simulink model "VTOLAutopilotController (minhyun-purdue's conflicted copy 2025-07-07)"  (R2024b)
settings: configuration reference "VTOLConfiguration" (kept outside this file)
undefined symbols (not defined in the file): control, controlParams, ControlSampleTime, CriticalTiltAngle, DiscIntNeverNeededParam, dspblkCoreblockFVToolHelper, flightState, FSState, FWControlParams, FWTrimSpeed, gcbh, HoverMission, R_LOOKAHEAD, ReferenceFilterDen, ReferenceFilterNum, tilt_max, tiltIni, uavParam, VTOLcontrolGains, w_trim, WindDownRate
libraries: slpidlib x32, simulink x11, uavalgslib x7, simulink_extras x1
(part 1 of 6)
settings Model: DataDictionary=VTOLDynamicsData.sldd  Creator=The MathWorks, Inc.  LastModifiedBy=mhcho
settings ConfigSetRef: SourceName=VTOLConfiguration

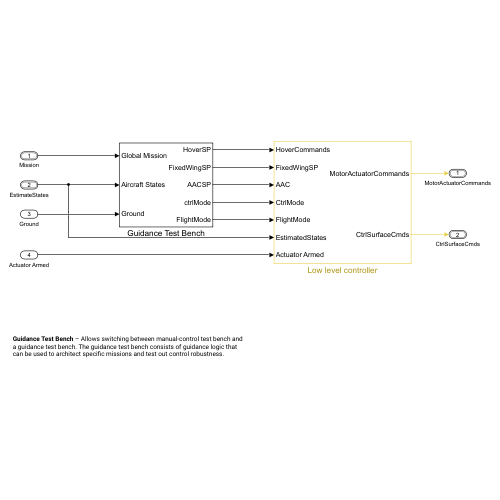
[thumbnail: Simulink's stored preview of the top-level diagram]
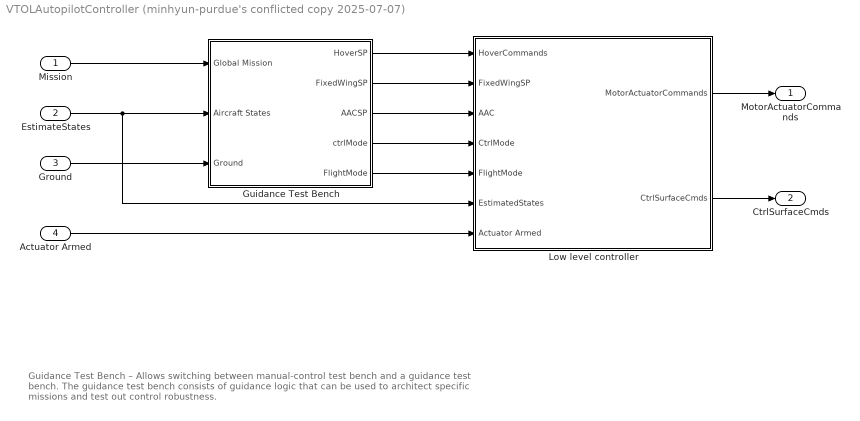
== system VTOLAutopilotController (minhyun-purdue's conflicted copy 2025-07-07) ==
  note: Guidance Test Bench – Allows switching between manual-control test bench and a guidance test bench. The guidance test bench consists of guidance logic that can be used to architect specific missions and test out control robustness.
  Mission : Inport  OutDataTypeStr=Bus: doubleUavPathManager  PortDimensions=length(HoverMission)  SampleTime=0.005  BusOutputAsStruct=on
  EstimateStates : Inport  Port=2  OutDataTypeStr=Bus: stateBus  BusOutputAsStruct=on
  Ground : Inport  Port=3  SampleTime=0.005
  Actuator Armed : Inport  Port=4
  Guidance Test Bench : Subsystem
  Low level controller : Subsystem
  MotorActuatorCommands : Outport  OutDataTypeStr=Bus: RotorCtrlBus  BusOutputAsStruct=on
  CtrlSurfaceCmds : Outport  Port=2  OutDataTypeStr=Bus: FixedWingCtrlBus  BusOutputAsStruct=on
  wires:
  Guidance Test Bench/1(HoverSP) -> Low level controller/1(HoverCommands)
  Guidance Test Bench/3(AACSP) -> Low level controller/3(AAC)
  Guidance Test Bench/5(FlightMode) -> Low level controller/5(FlightMode)
  Guidance Test Bench/4(ctrlMode) -> Low level controller/4(CtrlMode)
  EstimateStates/1 -> Guidance Test Bench/2(Aircraft States), Low level controller/6(EstimatedStates)
  Low level controller/1(MotorActuatorCommands) -> MotorActuatorCommands/1
  Mission/1 -> Guidance Test Bench/1(Global Mission)
  Guidance Test Bench/2(FixedWingSP) -> Low level controller/2(FixedWingSP)
  Low level controller/2(CtrlSurfaceCmds) -> CtrlSurfaceCmds/1
  Ground/1 -> Guidance Test Bench/3(Ground)
  Actuator Armed/1 -> Low level controller/7(Actuator Armed)

== system VTOLAutopilotController (minhyun-purdue's conflicted copy 2025-07-07)/Guidance Test Bench ==
  note: Set control type. In the project shortcut, choose between:
      | 1. Manual control by selecting Manual Mode under Hover and open the subsystem to manually control the UAV in hover mode.
      | 2. Guidance testbench with prebuilt mission by selecting Guidance Mod e in the project shortcut.
  Global Mission : Inport
  Aircraft States : Inport  Port=2
  Ground : Inport  Port=3
  ControlType : Subsystem  Variant=on  VariantControl=Choice
  Variant Subsystem : Subsystem  Variant=on
      settings: PortSchema="{\"entries\":[{\"content\":{\"sides\":[{\"content\":{\"connectorIds\":[\"In1\"]},\"type\":\"ConnectorPlacement.EquallySpacedRectSide\",\"uuid\":\"9fdb7eb7-bc98-4ae8-8dfe-5c3a3cbe5bd4\"},{\"content\":{\"connectorIds\":[\"In2\",\"In3\"],\"side\":\"RIGHT\"},\"type\":\"ConnectorPlacement.EquallySpacedRectSide\",\"uuid\":\"6c20d813-5cc1-435b-898c-bc09e61a7ed0\"},{\"content\":{\"side\":\"TOP\"},\"type\":\"ConnectorPlacement.EquallySpacedRectSide\",\"uuid\":\"a99c14f5-f5c7-4b02-b3e4-43ca7266f03f\"}]},\"type\":\"ConnectorPlacement.EquallySpacedConnector\",\"uuid\":\"e822b786-0a0c-436e-b41c-201e2beca970\"}],\"packageUris\":[\"http://schema.mathworks.com/mf0/Connector/R2020b\"],\"version\":\"1.0\"}"
  HoverSP : Outport
  FixedWingSP : Outport  Port=2
  AACSP : Outport  Port=3
  ctrlMode : Outport  Port=4
  FlightMode : Outport  Port=5
  wires:
  ControlType/1(HoverCmds) -> Variant Subsystem/2(Position), HoverSP/1
  Global Mission/1 -> ControlType/2(Global Mission)
  ControlType/2(FixedWingSP) -> FixedWingSP/1
  ControlType/5(FlightMode) -> FlightMode/1
  ControlType/4(ctrlMode) -> ctrlMode/1
  ControlType/3(AACSP) -> Variant Subsystem/3(AAC), AACSP/1
  Aircraft States/1 -> Variant Subsystem/1(State), ControlType/1(Aircraft States)
  Ground/1 -> ControlType/3(Ground)

== system VTOLAutopilotController (minhyun-purdue's conflicted copy 2025-07-07)/Low level controller ==
  HoverCommands : Inport
  FixedWingSP : Inport  Port=2
  AAC : Inport  Port=3
  CtrlMode : Inport  Port=4
  FlightMode : Inport  Port=5
  EstimatedStates : Inport  Port=6
  Actuator Armed : Inport  Port=7
  Bus Selector : BusSelector  OutputSignals=inTransition
  Bus Selector1 : BusSelector  OutputSignals=TransitionCondition
  Filter or Estimator : Subsystem
  Fixed Wing Controller : Subsystem  TreatAsAtomicUnit=on  VariantControl=Fixed Wing Controller
  Manual Control : Subsystem
  Multicopter Controller : Subsystem  TreatAsAtomicUnit=on
  Scheduler : Subsystem  SystemSampleTime=0.005
  Tilt Scheduler : Subsystem
  MotorActuatorCommands : Outport
  CtrlSurfaceCmds : Outport  Port=2
  wires:
  EstimatedStates/1 -> Filter or Estimator/1(SensorData)
  [TransitionDone] -> Scheduler/4(TransitionDone)
  Bus Selector1/1 -> [TransitionDone]  "<TransitionCondition>"
  Filter or Estimator/1(States) -> Scheduler/5(States), Multicopter Controller/2(States), Tilt Scheduler/2(States), Fixed Wing Controller/1(States)
  Scheduler/1(MotorActuatorCommands) -> MotorActuatorCommands/1
  Scheduler/2(CtrlSurfaceCommands) -> CtrlSurfaceCmds/1
  FlightMode/1 -> Multicopter Controller/4(FlightMode), Tilt Scheduler/1(FlightMode)
  HoverCommands/1 -> Multicopter Controller/1(Hover Commands)
  Manual Control/1(AERT) -> Fixed Wing Controller/5(AERT)
  Tilt Scheduler/2(FlightState) -> Scheduler/3(FlightState)
  Tilt Scheduler/1(TiltAngle) -> Scheduler/2(TiltSchedule)
  AAC/1 -> Fixed Wing Controller/3(AAC SP)
  CtrlMode/1 -> Fixed Wing Controller/2(Control Mode), Bus Selector1/1, Bus Selector/1
  Actuator Armed/1 -> Scheduler/Enable, Fixed Wing Controller/Enable, Multicopter Controller/Enable
  FixedWingSP/1 -> Fixed Wing Controller/4(FixedWingSP)
  Multicopter Controller/1(MixerCommands) -> Scheduler/1(MotorCommands)
  Bus Selector/1 -> Multicopter Controller/3(InTransition)  "<inTransition>"
  Fixed Wing Controller/1(Actuator) -> Scheduler/6(FixedWingActuators)

== system VTOLAutopilotController (minhyun-purdue's conflicted copy 2025-07-07)/Guidance Test Bench/ControlType ==
  Aircraft States : Inport
  Global Mission : Inport  Port=2
  Ground : Inport  Port=3
  Guidance Testbench : Subsystem  TreatAsAtomicUnit=on  VariantControl=TestMode==1
  Manual Control : Subsystem  TreatAsAtomicUnit=on  VariantControl=TestMode==0
  HoverCmds : Outport
  FixedWingSP : Outport  Port=2
  AACSP : Outport  Port=3
  ctrlMode : Outport  Port=4
  FlightMode : Outport  Port=5

== system VTOLAutopilotController (minhyun-purdue's conflicted copy 2025-07-07)/Guidance Test Bench/Variant Subsystem ==
  note: 1) Add Subsystem or Model blocks as valid variant choices.
      | 2) You cannot connect blocks at this level. At simulation, connectivity is automatically
      | determined, based on the active variant and port name matching.
  State : Inport
  Position : Inport  Port=2
  AAC : Inport  Port=3
  No-op : Subsystem  VariantControl=Deployment == true
  "Reference Tracking " : Subsystem  VariantControl=Deployment == false

== system VTOLAutopilotController (minhyun-purdue's conflicted copy 2025-07-07)/Low level controller/Filter or Estimator ==
  SensorData : Inport
  States : Outport
  wires:
  SensorData/1 -> States/1

== system VTOLAutopilotController (minhyun-purdue's conflicted copy 2025-07-07)/Low level controller/Fixed Wing Controller ==
  States : Inport
  Control Mode : Inport  Port=2
  AAC SP : Inport  Port=3
  FixedWingSP : Inport  Port=4
  AERT : Inport  Port=5
  Enable : EnablePort
  Fixed Wing Controller Module : Subsystem  Variant=on  VariantControl=TuningMode == 0
  Actuator : Outport
  wires:
  States/1 -> Fixed Wing Controller Module/1(States)
  Control Mode/1 -> Fixed Wing Controller Module/2(Control Mode)
  AAC SP/1 -> Fixed Wing Controller Module/3(AAC SP)
  FixedWingSP/1 -> Fixed Wing Controller Module/4(FixedWingSP)
  AERT/1 -> Fixed Wing Controller Module/5(AERT)
  Fixed Wing Controller Module/1(Actuator) -> Actuator/1

== system VTOLAutopilotController (minhyun-purdue's conflicted copy 2025-07-07)/Low level controller/Manual Control ==
  Bus Creator : BusCreator  Inputs=4
  Constant{,1..3} (4 alike) : Constant  Value=0  SampleTime=-1
  AERT : Outport
  wires:
  Constant/1 -> Bus Creator/1  "aileron"
  Constant1/1 -> Bus Creator/2  "throttle"
  Constant2/1 -> Bus Creator/3  "elevator"
  Constant3/1 -> Bus Creator/4  "rudder"
  Bus Creator/1 -> AERT/1

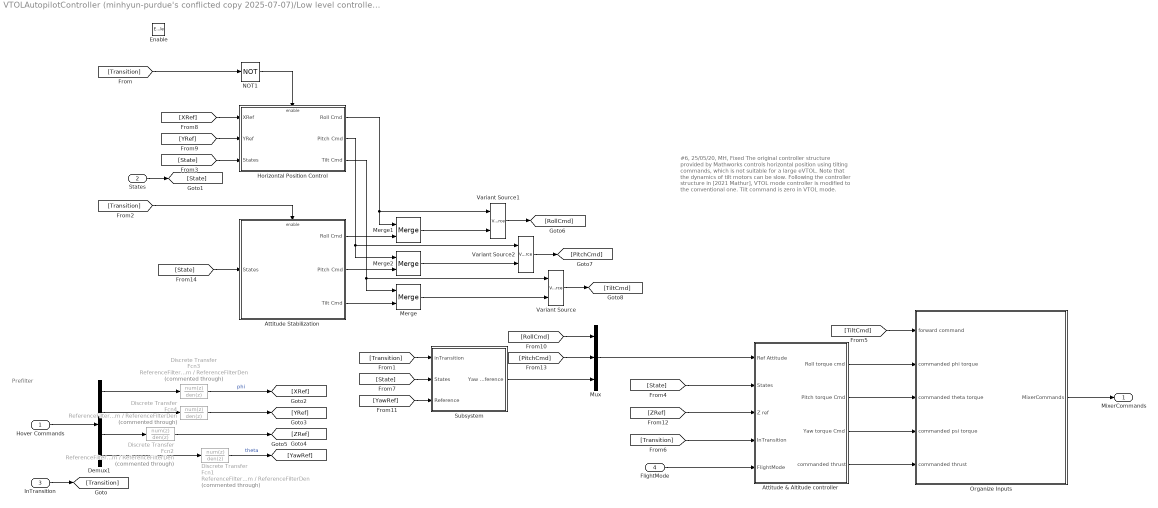
== system VTOLAutopilotController (minhyun-purdue's conflicted copy 2025-07-07)/Low level controller/Multicopter Controller ==
  note: Prefilter
  note: #6, 25/05/20, MH, Fixed
      | The original controller structure provided by
      | Mathworks controls horizontal position using
      | tilting commands, which is not suitable for
      | a large eVTOL. Note that the dynamics of tilt
      | motors can be slow. Following the controller
      | structure in [2021 Mathur], VTOL mode controller
      | is modified to the conventional one.
      | Tilt command is zero in VTOL mode.
  Hover Commands : Inport
  States : Inport  Port=2
  InTransition : Inport  Port=3
  FlightMode : Inport  Port=4
  Enable : EnablePort
  Attitude & Altitude controller : Subsystem
  Attitude Stabilization : Subsystem  TreatAsAtomicUnit=on
  Demux1 : Demux
  Discrete Transfer Fcn1 : DiscreteTransferFcn  Commented=through  LoadFcn=dspblkCoreblockFVToolHelper(gcbh,'load');  Numerator=ReferenceFilterNum  Denominator=ReferenceFilterDen
      settings: CopyFcn=dspblkCoreblockFVToolHelper(gcbh,'copy');  DeleteFcn=dspblkCoreblockFVToolHelper(gcbh,'close');  ModelCloseFcn=dspblkCoreblockFVToolHelper(gcbh,'close');  PreSaveFcn=dspblkCoreblockFVToolHelper(gcbh,'presave');  PostSaveFcn=dspblkCoreblockFVToolHelper(gcbh,'postsave');  CloseFcn=dspblkCoreblockFVToolHelper(gcbh,'close');
  Discrete Transfer Fcn2 : DiscreteTransferFcn  Commented=through  Numerator=ReferenceFilterNum  Denominator=ReferenceFilterDen
  Discrete Transfer Fcn3 : DiscreteTransferFcn  Commented=through  Numerator=ReferenceFilterNum  Denominator=ReferenceFilterDen
  Discrete Transfer Fcn4 : DiscreteTransferFcn  Commented=through  Numerator=ReferenceFilterNum  Denominator=ReferenceFilterDen
  Horizontal Position Control : Subsystem  TreatAsAtomicUnit=on
  Merge : Merge
  Merge1 : Merge
  Merge2 : Merge
  Mux : Mux  Inputs=3
  NOT1 : Logic  Operator=NOT  IconShape=distinctive  AllPortsSameDT=off  OutDataTypeStr=boolean
  Organize Inputs : Subsystem
  Subsystem : Subsystem
  Variant Source : VariantSource
  Variant Source1 : VariantSource
  Variant Source2 : VariantSource
  MixerCommands : Outport
  wires:
  Organize Inputs/1(MixerCommands) -> MixerCommands/1
  [State] -> Subsystem/2(States)
  Discrete Transfer Fcn4/1 -> [YRef]
  Demux1/1 -> Discrete Transfer Fcn3/1
  [State] -> Horizontal Position Control/3(States)
  Demux1/2 -> Discrete Transfer Fcn4/1
  Attitude Stabilization/3(Tilt Cmd) -> Merge/2
  [YawRef] -> Subsystem/3(Reference)
  Merge/1 -> Variant Source/2
  Merge1/1 -> Variant Source1/2
  [Transition] -> Subsystem/1(inTransition)
  Demux1/3 -> Discrete Transfer Fcn2/1
  Attitude Stabilization/1(Roll Cmd) -> Merge1/2
  Horizontal Position Control/1(Roll Cmd) -> Merge1/1, Variant Source1/1
  [Transition] -> Attitude Stabilization/Enable
  NOT1/1 -> Horizontal Position Control/Enable
  Discrete Transfer Fcn2/1 -> [ZRef]
  [XRef] -> Horizontal Position Control/1(XRef)
  [YRef] -> Horizontal Position Control/2(YRef)
  InTransition/1 -> [Transition]
  States/1 -> [State]
  Horizontal Position Control/3(Tilt Cmd) -> Variant Source/1, Merge/1
  Hover Commands/1 -> Demux1/1
  Demux1/4 -> Discrete Transfer Fcn1/1
  Mux/1 -> Attitude & Altitude controller/1(Ref Attitude)
  [State] -> Attitude & Altitude controller/2(States)
  [ZRef] -> Attitude & Altitude controller/3(Z ref)
  [Transition] -> Attitude & Altitude controller/4(InTransition)
  Attitude & Altitude controller/1(Roll torque cmd) -> Organize Inputs/2(commanded phi torque)
  Attitude & Altitude controller/2(Pitch torque Cmd) -> Organize Inputs/3(commanded theta torque)
  Attitude & Altitude controller/4(commanded thrust) -> Organize Inputs/5(commanded thrust)
  FlightMode/1 -> Attitude & Altitude controller/5(FlightMode)
  Discrete Transfer Fcn3/1 -> [XRef]  "phi"
  Attitude & Altitude controller/3(Yaw torque Cmd) -> Organize Inputs/4(commanded psi torque)
  Discrete Transfer Fcn1/1 -> [YawRef]  "theta"
  [Transition] -> NOT1/1
  Attitude Stabilization/2(Pitch Cmd) -> Merge2/2
  Horizontal Position Control/2(Pitch Cmd) -> Merge2/1, Variant Source2/1
  Variant Source1/1 -> [RollCmd]
  Variant Source2/1 -> [PitchCmd]
  Merge2/1 -> Variant Source2/2
  Variant Source/1 -> [TiltCmd]
  [TiltCmd] -> Organize Inputs/1(forward command)
  [RollCmd] -> Mux/1
  [PitchCmd] -> Mux/2
  Subsystem/1(Yaw Reference) -> Mux/3
  [State] -> Attitude Stabilization/1(States)

== system VTOLAutopilotController (minhyun-purdue's conflicted copy 2025-07-07)/Low level controller/Scheduler ==
  MotorCommands : Inport
  TiltSchedule : Inport  Port=2
  FlightState : Inport  Port=3  OutDataTypeStr=Enum: flightState
  TransitionDone : Inport  Port=4
  States : Inport  Port=5
  FixedWingActuators : Inport  Port=6
  Enable : EnablePort
  FixedWingScheduler : Subsystem
  Subsystem : Subsystem
  MotorActuatorCommands : Outport  OutputWhenDisabled=reset  InitialOutput=0
  CtrlSurfaceCommands : Outport  Port=2  OutDataTypeStr=Bus: FixedWingCtrlBus  OutputWhenDisabled=reset  InitialOutput=0  VectorParamsAs1DForOutWhenUnconnected=off
  wires:
  FixedWingScheduler/1(ActuatorControls) -> Subsystem/2(FixedWingActuators), CtrlSurfaceCommands/1
  FlightState/1 -> [FlightState], FixedWingScheduler/1(FlightState)
  TiltSchedule/1 -> Subsystem/4(TiltSchedule)
  Subsystem/1(ActuatorControls) -> MotorActuatorCommands/1
  MotorCommands/1 -> Subsystem/3(MotorCommands)
  FixedWingActuators/1 -> FixedWingScheduler/2(FixedWingActuators)
  TransitionDone/1 -> FixedWingScheduler/3(TransitionDone), [TransitionDone]
  States/1 -> Subsystem/6(States)
  [FlightState] -> Subsystem/1(FlightState)
  [TransitionDone] -> Subsystem/5(TransitionDone)

== system VTOLAutopilotController (minhyun-purdue's conflicted copy 2025-07-07)/Low level controller/Tilt Scheduler ==
  note: Forward Transition Tilt Mode Manager
  note: Back Transition Tilt Mode Manager
  FlightMode : Inport
  States : Inport  Port=2
  Back Transition Scheduler : Subsystem
  Forward Transition Scheduler : Subsystem
  TiltAngle : Outport
  FlightState : Outport  Port=2
  wires:
  States/1 -> Back Transition Scheduler/3(States)
  Back Transition Scheduler/1(TiltAngle) -> TiltAngle/1
  FlightMode/1 -> Back Transition Scheduler/2(FlightMode), Forward Transition Scheduler/1(FlightMode)
  Forward Transition Scheduler/1(FlightState) -> FlightState/1
  Forward Transition Scheduler/2(Tilt Schedule) -> Back Transition Scheduler/1(Tilt Schedule)

== system VTOLAutopilotController (minhyun-purdue's conflicted copy 2025-07-07)/Guidance Test Bench/ControlType/Guidance Testbench ==
  Global Mission : Inport
  Aircraft States : Inport  Port=2
  Ground : Inport  Port=3
  Control Rate Transition : Subsystem
  Guidance Logic : Subsystem  VariantControl=guidanceType==1
  HoverCmds : Outport
  FixedWingSP : Outport  Port=2
  AACSP : Outport  Port=3
  ctrlMode : Outport  Port=4
  FlightMode : Outport  Port=5
  wires:
  Aircraft States/1 -> Guidance Logic/1(UAVState)
  Global Mission/1 -> Guidance Logic/2(GCSCommands)
  Guidance Logic/1(HoverGuidance) -> Control Rate Transition/1("1 ")
  Guidance Logic/2(FixedWingSP) -> Control Rate Transition/2(In2)
  Guidance Logic/3(AACSP) -> Control Rate Transition/3(In3)
  Guidance Logic/4(ctrlMode) -> Control Rate Transition/4(In4)
  Guidance Logic/5(FlightMode) -> Control Rate Transition/5(In5)
  Control Rate Transition/1(Out1) -> HoverCmds/1
  Control Rate Transition/2(Out2) -> FixedWingSP/1
  Control Rate Transition/3(Out3) -> AACSP/1
  Control Rate Transition/4(Out4) -> ctrlMode/1
  Control Rate Transition/5(Out5) -> FlightMode/1
  Ground/1 -> Guidance Logic/3(Ground)

== system VTOLAutopilotController (minhyun-purdue's conflicted copy 2025-07-07)/Guidance Test Bench/ControlType/Manual Control ==
  Global Mission : Inport
  Aircraft States : Inport  Port=2
  Command Interface : Subsystem
  HoverCmds : Outport
  FixedWingSP : Outport  Port=2
  AACSP : Outport  Port=3
  ctrlMode : Outport  Port=4
  FlightMode : Outport  Port=5
  wires:
  Global Mission/1 -> Command Interface/1(Global Mission)
  Aircraft States/1 -> Command Interface/2(Aircraft States)
  Command Interface/1(ctrlMode) -> ctrlMode/1
  Command Interface/2(FixedWingSP) -> FixedWingSP/1
  Command Interface/3(AACSP) -> AACSP/1
  Command Interface/4(PositionCmds) -> HoverCmds/1
  Command Interface/5(FlightMode) -> FlightMode/1

== system VTOLAutopilotController (minhyun-purdue's conflicted copy 2025-07-07)/Guidance Test Bench/Variant Subsystem/No-op ==
  State : Inport
  Terminator : Terminator
  wires:
  State/1 -> Terminator/1

== system VTOLAutopilotController (minhyun-purdue's conflicted copy 2025-07-07)/Guidance Test Bench/Variant Subsystem/Reference Tracking  ==
  State : Inport
  Position : Inport  Port=2
  AAC : Inport  Port=3
  Fixed Wing Reference : Subsystem
  Hover Reference : Subsystem
  Transition Reference : Subsystem
  wires:
  State/1 -> Transition Reference/1(States), Fixed Wing Reference/2(States), Hover Reference/2(Position Reference)
  AAC/1 -> Fixed Wing Reference/1(AAC Commands)
  Position/1 -> Hover Reference/1(Position Command)

== system VTOLAutopilotController (minhyun-purdue's conflicted copy 2025-07-07)/Low level controller/Fixed Wing Controller/Fixed Wing Controller Module ==
  States : Inport
  Control Mode : Inport  Port=2
  AAC SP : Inport  Port=3
  FixedWingSP : Inport  Port=4
  AERT : Inport  Port=5
  Fixed Wing Controller Simulation : Subsystem  VariantControl=TuningMode == 0
  Fixed Wing Controller Tuning : Subsystem  VariantControl=TuningMode==1
  Actuator : Outport

== system VTOLAutopilotController (minhyun-purdue's conflicted copy 2025-07-07)/Low level controller/Multicopter Controller/Attitude & Altitude controller ==
  Ref Attitude : Inport
  States : Inport  Port=2
  Z ref : Inport  Port=3
  InTransition : Inport  Port=4
  FlightMode : Inport  Port=5
  Altitude Control : Subsystem
      settings: PortSchema="{\"entries\":[{\"content\":{\"sides\":[{\"content\":{\"connectorIds\":[\"In1\",\"In2\",\"In3\"]},\"type\":\"ConnectorPlacement.EquallySpacedRectSide\",\"uuid\":\"0fb78ff2-45dd-421f-94dd-13101ee8437b\"},{\"content\":{\"connectorIds\":[\"Out1\"],\"side\":\"RIGHT\"},\"type\":\"ConnectorPlacement.EquallySpacedRectSide\",\"uuid\":\"b9be60f2-cff5-482a-9939-1f361dc87644\"},{\"content\":{\"side\":\"TOP\"},\"type\":\"ConnectorPlacement.EquallySpacedRectSide\",\"uuid\":\"5554a5d5-69cd-48ac-8e70-482785654dbe\"},{\"content\":{\"connectorIds\":[\"In4\"],\"side\":\"BOTTOM\"},\"type\":\"ConnectorPlacement.EquallySpacedRectSide\",\"uuid\":\"0845aa0b-84ad-4767-a072-4aa91dc150b4\"}]},\"type\":\"ConnectorPlacement.EquallySpacedConnector\",\"uuid\":\"b37117b5-baa1-4c31-85d5-a94c3f794c14\"}],\"packageUris\":[\"http://schema.mathworks.com/mf0/Connector/R2020b\"],\"version\":\"1.0\"}"
  Derivative Gain : Subsystem  VariantControl=AttitudeControl==1
  Roll torque cmd : Outport
  Pitch torque Cmd : Outport  Port=2
  Yaw torque Cmd : Outport  Port=3
  commanded thrust : Outport  Port=4
  wires:
  Altitude Control/1(commanded thrust) -> commanded thrust/1
  Derivative Gain/1(Roll torque cmd) -> Roll torque cmd/1
  InTransition/1 -> Altitude Control/3(InTransition)
  Derivative Gain/2(Pitch torque Cmd) -> Pitch torque Cmd/1
  States/1 -> Altitude Control/1(States), Derivative Gain/2(States)
  Derivative Gain/3(Yaw torque Cmd) -> Yaw torque Cmd/1
  Z ref/1 -> Altitude Control/2(Z ref)
  FlightMode/1 -> Altitude Control/4(FlightMode)
  Ref Attitude/1 -> Derivative Gain/1(Ref Attitude)

== system VTOLAutopilotController (minhyun-purdue's conflicted copy 2025-07-07)/Low level controller/Multicopter Controller/Attitude Stabilization ==
  note: Level Tiltrotor when in transition.
  note: #TODO, 25/07/05, MH, Not Fixed
      | Use this for backward transition.
  States : Inport
  Enable : EnablePort
  Bus Selector : BusSelector  OutputSignals=Euler,Ve
  Constant{,1..3} (4 alike) : Constant  Value=0
  Forward velocity : Subsystem
  Selector : Selector  InputPortWidth=3  IndexOptions=Index vector (dialog)  Indices=[3]  OutputSizes=1
  Selector1 : Selector  InputPortWidth=3  IndexOptions=Index vector (dialog)  Indices=[2]  OutputSizes=1
  Selector2 : Selector  InputPortWidth=3  IndexOptions=Index vector (dialog)  Indices=[1]  OutputSizes=1
  SinCos : Trigonometry  Operator=sincos
  Sum3 : Sum  Inputs=+-
  Terminator : Terminator
  Roll Cmd : Outport
  Pitch Cmd : Outport  Port=2
  Tilt Cmd : Outport  Port=3
  wires:
  Constant/1 -> Tilt Cmd/1
  Constant1/1 -> Roll Cmd/1
  Constant2/1 -> Pitch Cmd/1
  Bus Selector/1 -> Selector/1  "<Euler>"
  Selector/1 -> SinCos/1  "yaw"
  States/1 -> Bus Selector/1
  Bus Selector/2 -> Selector2/1, Selector1/1  "<Ve>"
  Selector1/1 -> Forward velocity/1(vy)
  Selector2/1 -> Forward velocity/2(vx)
  SinCos/1 -> Forward velocity/3(sin)
  SinCos/2 -> Forward velocity/4(cos)
  Constant3/1 -> Sum3/1
  Forward velocity/1(ef) -> Sum3/2  "vf"
  Sum3/1 -> Terminator/1

== system VTOLAutopilotController (minhyun-purdue's conflicted copy 2025-07-07)/Low level controller/Multicopter Controller/Horizontal Position Control ==
  note: Forward Motion is controlled using Tilt.
      | Lateral Motion occurs using roll.
  XRef : Inport
  YRef : Inport  Port=2
  States : Inport  Port=3
  Enable : EnablePort
  Constant : Constant  Value=0
  Gain : Gain  Gain=-1
  Rate Limiter : RateLimiter  RisingSlewLimit=5.1  FallingSlewLimit=-5.1  SampleTimeMode=inherited
  Rate Limiter1 : RateLimiter  RisingSlewLimit=5.1  FallingSlewLimit=-5.1  SampleTimeMode=inherited
  Saturation : Saturate  UpperLimit=0.25  LowerLimit=-0.25
  Saturation1 : Saturate  UpperLimit=30/180*pi  LowerLimit=-30/180*pi
  XY Controller : Subsystem
  Roll Cmd : Outport
  Pitch Cmd : Outport  Port=2
  Tilt Cmd : Outport  Port=3
  wires:
  XRef/1 -> XY Controller/1(X_ref)
  YRef/1 -> XY Controller/2(Y_ref)
  States/1 -> XY Controller/3(States)
  XY Controller/1(Forward cmd) -> Saturation1/1
  XY Controller/2(Sideward Cmd) -> Saturation/1
  Saturation/1 -> Rate Limiter/1
  Rate Limiter/1 -> Roll Cmd/1
  Saturation1/1 -> Rate Limiter1/1
  Constant/1 -> Tilt Cmd/1
  Gain/1 -> Pitch Cmd/1
  Rate Limiter1/1 -> Gain/1

== system VTOLAutopilotController (minhyun-purdue's conflicted copy 2025-07-07)/Low level controller/Multicopter Controller/Organize Inputs ==
  forward command : Inport
  commanded phi torque : Inport  Port=2
  commanded theta torque : Inport  Port=3
  commanded psi torque : Inport  Port=4
  commanded thrust : Inport  Port=5
  Out Bus Element : Outport  PortName=MixerCommands  Element=w_phi
  Out Bus Element1 : Outport  PortName=MixerCommands  Element=w_theta
  Out Bus Element2 : Outport  PortName=MixerCommands  Element=w_psi
  Out Bus Element3 : Outport  PortName=MixerCommands  Element=w_z
  Out Bus Element4 : Outport  PortName=MixerCommands  Element=l_x
  tag scope: w_phi=global, w_psi=global, w_theta=global, w_tilt=global, w_z=global
  wires:
  commanded theta torque/1 -> [w_theta], Out Bus Element1/1  "theta"
  commanded psi torque/1 -> Out Bus Element2/1, [w_psi]
  commanded thrust/1 -> [w_z], Out Bus Element3/1
  forward command/1 -> Out Bus Element4/1, [w_tilt]
  commanded phi torque/1 -> Out Bus Element/1, [w_phi]  "phi"

== system VTOLAutopilotController (minhyun-purdue's conflicted copy 2025-07-07)/Low level controller/Multicopter Controller/Subsystem ==
  inTransition : Inport
  States : Inport  Port=2
  Reference : Inport  Port=3
  Bus Selector : BusSelector  OutputSignals=ypr
  NOT : Logic  Operator=NOT  IconShape=distinctive  AllPortsSameDT=off  OutDataTypeStr=boolean
  Selector : Selector  InputPortWidth=3  IndexOptions=Index vector (dialog)  Indices=[1]  OutputSizes=1
  Switch : Switch  Criteria=u2 > Threshold  SaturateOnIntegerOverflow=off  InputSameDT=off
  Triggered Subsystem : Subsystem  TreatAsAtomicUnit=on
  Yaw Reference : Outport
  wires:
  inTransition/1 -> NOT/1, Triggered Subsystem/Trigger
  States/1 -> Bus Selector/1
  Bus Selector/1 -> Selector/1  "<ypr>"
  Selector/1 -> Triggered Subsystem/1(YawHold)
  NOT/1 -> Switch/2
  Triggered Subsystem/1(Reference) -> Switch/3  "Stable"
  Switch/1 -> Yaw Reference/1
  Reference/1 -> Switch/1

== system VTOLAutopilotController (minhyun-purdue's conflicted copy 2025-07-07)/Low level controller/Scheduler/FixedWingScheduler ==
  note: C opyright 2024 The MathWorks, Inc.
  note: Fixed Wing Control Mixer
  FlightState : Inport
  FixedWingActuators : Inport  Port=2  OutDataTypeStr=Bus: FixedWingCtrlBus
  TransitionDone : Inport  Port=3
  Merge : Merge  Inputs=4
  Switch Case : SwitchCase  CaseConditions={flightState.Hover, flightState.Transition, flightState.FixedWing,flightState.BackTransition}  ShowDefaultCase=off
  Switch Case Action Subsystem : Subsystem  TreatAsAtomicUnit=on
  Switch Case Action Subsystem1 : Subsystem  TreatAsAtomicUnit=on
  Switch Case Action Subsystem2 : Subsystem  TreatAsAtomicUnit=on
  Switch Case Action Subsystem3 : Subsystem  TreatAsAtomicUnit=on
  ActuatorControls : Outport
  wires:
  FlightState/1 -> Switch Case/1
  FixedWingActuators/1 -> Switch Case Action Subsystem2/1(FixedWingActuators), Switch Case Action Subsystem1/1(FixedWingActuators)
  Switch Case/3 -> Switch Case Action Subsystem2/Action
  Switch Case/2 -> Switch Case Action Subsystem1/Action
  TransitionDone/1 -> Switch Case Action Subsystem1/2(TransitionDone)
  Switch Case Action Subsystem3/1(FixedWingControls) -> Merge/4
  Merge/1 -> ActuatorControls/1
  Switch Case Action Subsystem1/1(FixedWingControls) -> Merge/2
  Switch Case/4 -> Switch Case Action Subsystem3/Action
  Switch Case Action Subsystem/1(FixedWingControls) -> Merge/1
  Switch Case/1 -> Switch Case Action Subsystem/Action
  Switch Case Action Subsystem2/1(FixedWingControls) -> Merge/3

== system VTOLAutopilotController (minhyun-purdue's conflicted copy 2025-07-07)/Low level controller/Scheduler/Subsystem ==
  note: C opyright 2024 The MathWorks, Inc.
  note: Multicopter Control Mixer
  FlightState : Inport
  FixedWingActuators : Inport  Port=2
  MotorCommands : Inport  Port=3
  TiltSchedule : Inport  Port=4
  TransitionDone : Inport  Port=5
  States : Inport  Port=6
  Actuator To Voltage : Subsystem
  Merge : Merge  Inputs=4
  Switch Case : SwitchCase  CaseConditions={flightState.Hover, flightState.Transition, flightState.FixedWing,flightState.BackTransition}  ShowDefaultCase=off
  Switch Case Action Subsystem : Subsystem  TreatAsAtomicUnit=on
  Switch Case Action Subsystem1 : Subsystem  TreatAsAtomicUnit=on
  Switch Case Action Subsystem2 : Subsystem  TreatAsAtomicUnit=on
  Switch Case Action Subsystem3 : Subsystem  TreatAsAtomicUnit=on
  ActuatorControls : Outport  OutDataTypeStr=Bus: RotorCtrlBus
  wires:
  Merge/1 -> Actuator To Voltage/1(Motor Commands)
  Switch Case/4 -> Switch Case Action Subsystem3/Action
  MotorCommands/1 -> Switch Case Action Subsystem3/1(MixerCommands), Switch Case Action Subsystem1/2(MixerCommands), Switch Case Action Subsystem/1(MixerCommands)
  States/1 -> Switch Case Action Subsystem1/5(State), Switch Case Action Subsystem2/3(State)
  Switch Case Action Subsystem2/1(Actuator) -> Merge/3
  FlightState/1 -> Switch Case/1
  Switch Case Action Subsystem/1(Actuator) -> Merge/1
  Switch Case Action Subsystem3/1(Actuator) -> Merge/4
  FixedWingActuators/1 -> Switch Case Action Subsystem2/1(FixedWingCtrlBus), Switch Case Action Subsystem1/3(FixedWing)
  Switch Case/3 -> Switch Case Action Subsystem2/Action
  TransitionDone/1 -> Switch Case Action Subsystem2/2(TransitionDone), Switch Case Action Subsystem1/4(TransitionDone)
  Actuator To Voltage/1(To PWM) -> ActuatorControls/1
  Switch Case/2 -> Switch Case Action Subsystem1/Action
  Switch Case Action Subsystem1/1(Actuator) -> Merge/2
  TiltSchedule/1 -> Switch Case Action Subsystem3/2(TiltSchedule), Switch Case Action Subsystem1/1(TiltSchedule)
  Switch Case/1 -> Switch Case Action Subsystem/Action

== system VTOLAutopilotController (minhyun-purdue's conflicted copy 2025-07-07)/Low level controller/Tilt Scheduler/Back Transition Scheduler ==
  Tilt Schedule : Inport
  FlightMode : Inport  Port=2
  States : Inport  Port=3
  Add : Sum  Inputs=+-
  Bus Selector : BusSelector  OutputSignals=Vb
  Constant1 : Constant  Value=flightState.BackTransition
  Constant6 : Constant  Value=4
  Equal1 : RelationalOperator  Operator===  OutDataTypeStr=boolean  RndMeth=Simplest  InputSameDT=off
  Saturation : Saturate  UpperLimit=pi/4  LowerLimit=-pi/4
  Scope : Scope
  Selector : Selector  InputPortWidth=3  IndexOptions=Index vector (dialog)  Indices=[1]  OutputSizes=1
  Switch2 : Switch  Threshold=1  SaturateOnIntegerOverflow=off  InputSameDT=off
  Vx Controller : slpidlib/PID Controller  Controller=P  Form=Parallel  TimeDomain=Discrete-time  UseExternalTs=off  SampleTime=0.005  IntegratorMethod=Forward Euler  FilterMethod=Forward Euler  ControllerParametersSource=internal  P=controlParams.P_BACK  I=0  UseKiTs=off  D=0.0379422021775223  UseExternalDerivativeSource=off  N=1.96946409823213  UseFilter=on  TunerSelectOption=Transfer Function Based (PID Tuner App)  InitialConditionSource=internal  InitialConditionForIntegrator=0  InitialConditionForFilter=0  DifferentiatorICPrevScaledInput=0  ExternalReset=none  TrackingMode=off  Kt=1  LimitOutput=off  SatLimitsSource=internal  UpperSaturationLimit=inf  LowerSaturationLimit=-inf  LinearizeAsGain=on  AntiWindupMode=none  Kb=1  LimitIntegrator=off  UpperIntegratorSaturationLimit=inf  LowerIntegratorSaturationLimit=-inf  POutMin=[]  POutMax=[]  IOutMin=[]  IOutMax=[]  DOutMin=[]  DOutMax=[]  NOutMin=[]  NOutMax=[]  SumOutMin=[]  SumOutMax=[]  SaturationOutMin=[]  SaturationOutMax=[]  PParamMin=[]  PParamMax=[]  IParamMin=[]  IParamMax=[]  DParamMin=[]  DParamMax=[]  NParamMin=[]  NParamMax=[]  KbParamMin=[]  KbParamMax=[]  KtParamMin=[]  KtParamMax=[]  KbOutMin=[]  KbOutMax=[]  KtOutMin=[]  KtOutMax=[]  IntegratorOutMin=[]  IntegratorOutMax=[]  FilterOutMin=[]  FilterOutMax=[]  SumI1OutMin=[]  SumI1OutMax=[]  SumI2OutMin=[]  SumI2OutMax=[]  SumI3OutMin=[]  SumI3OutMax=[]  SumI4OutMin=[]  SumI4OutMax=[]  SumDOutMin=[]  SumDOutMax=[]  DifferentiatorOutMin=[]  DifferentiatorOutMax=[]  FilterDiffOutCoefMin=[]  FilterDiffOutCoefMax=[]  ReciprocalOutMin=[]  ReciprocalOutMax=[]  SumDenOutMin=[]  SumDenOutMax=[]  SumNumOutMin=[]  SumNumOutMax=[]  DivideOutMin=[]  DivideOutMax=[]  UdiffTsProdOutMin=[]  UdiffTsProdOutMax=[]  NTsProdOutMin=[]  NTsProdOutMax=[]  UintegralTsProdOutMin=[]  UintegralTsProdOutMax=[]  UngainTsProdOutMin=[]  UngainTsProdOutMax=[]  ClampingZeroOutDataTypeStr=Inherit: Inherit via back propagation  ClampingZeroOutMin=[]  ClampingZeroOutMax=[]  FilterDenConstantOutDataTypeStr=Inherit: Inherit via back propagation  FilterDenConstantOutMin=[]  FilterDenConstantOutMax=[]  PCopyOutDataTypeStr=Inherit: Inherit via back propagation  PCopyOutMin=[]  PCopyOutMax=[]  NCopyOutDataTypeStr=Inherit: Inherit via back propagation  NCopyOutMin=[]  NCopyOutMax=[]  IntegratorContinuousStateAttributes=''  IntegratorStateMustResolveToSignalObject=off  IntegratorRTWStateStorageClass=Auto  FilterContinuousStateAttributes=''  FilterStateMustResolveToSignalObject=off  FilterRTWStateStorageClass=Auto  ParallelPVariant=InternalParameters  IdealPVariant=Disabled  IVariant=Disabled  DVariant=Disabled  IntegratorVariant=Disabled  SatVariant=Disabled  AWVariant=Disabled  PCopyVariant=Disabled  TRVariant=Disabled  FdbkBlocksVariant=Forward  IdealPFdbkVariant=Disabled  SatFdbkVariant=Disabled  DerivativeFilterVariant=Disabled  NVariant=Disabled  NCopyVariant=Disabled_SignalSpec  FilterICVariant=Disabled  IntegratorICVariant=Disabled  ExternalResetVariant=Disabled  TRSumVariant=Passthrough  SumFdbkVariant=Disabled  SumVariant=Passthrough_P  TsampFilterVariant=InternalTs  TsampNgainVariant=Passthrough  TsampIntegralVariant=Disabled_SignalSpec  ExternalSaturationOutDataTypeStr=Inherit: Same as second input  DerivativeSourceVariant=Disabled  PreIntVariant=InternalPreInt
  TiltAngle : Outport
  wires:
  States/1 -> Bus Selector/1
  Add/1 -> Vx Controller/1
  Equal1/1 -> Switch2/2
  Bus Selector/1 -> Selector/1  "<Vb>"
  FlightMode/1 -> Equal1/1
  Constant1/1 -> Equal1/2
  Constant6/1 -> Add/1
  Selector/1 -> Add/2
  Vx Controller/1 -> Saturation/1
  Saturation/1 -> Switch2/1
  Tilt Schedule/1 -> Switch2/3
  Switch2/1 -> Scope/1, TiltAngle/1

== system VTOLAutopilotController (minhyun-purdue's conflicted copy 2025-07-07)/Low level controller/Tilt Scheduler/Forward Transition Scheduler ==
  FlightMode : Inport
  Constant : Constant  Value=pi/2
  Constant2 : Constant  Value=0
  Constant3 : Constant  Value=controlParams.CriticalTiltAngle
  Constant4 : Constant  Value=flightState.Transition
  Constant5 : Constant  Value=controlParams.TiltScheduleRate
  Discrete-Time Integrator : DiscreteIntegrator  ExternalReset=either  SampleTime=-1  LimitOutput=on  LowerSaturationLimit=0  ICPrevOutput=DiscIntNeverNeededParam  ICPrevScaledInput=DiscIntNeverNeededParam
  Equal : RelationalOperator  Operator===  OutDataTypeStr=boolean  RndMeth=Simplest  InputSameDT=off
  LessThanOrEqual : RelationalOperator  Operator=<=  OutDataTypeStr=boolean  RndMeth=Simplest  InputSameDT=off
  Switch : Switch  Criteria=u2 > Threshold  SaturateOnIntegerOverflow=off  InputSameDT=off
  Switch1 : Switch  Criteria=u2 > Threshold  SaturateOnIntegerOverflow=off  InputSameDT=off
  FlightState : Outport
  Tilt Schedule : Outport  Port=2
  tag scope: ModeFlag=global
  wires:
  FlightMode/1 -> FlightState/1, Equal/2
  [ModeFlag] -> Discrete-Time Integrator/2, Switch1/2
  Discrete-Time Integrator/1 -> Switch/1, LessThanOrEqual/1
  LessThanOrEqual/1 -> Switch/2
  Equal/1 -> [ModeFlag]
  Constant3/1 -> LessThanOrEqual/2
  Switch1/1 -> Discrete-Time Integrator/1
  Constant5/1 -> Switch1/1
  Constant2/1 -> Switch1/3
  Constant4/1 -> Equal/1
  Constant/1 -> Switch/3
  Switch/1 -> Tilt Schedule/1

== system VTOLAutopilotController (minhyun-purdue's conflicted copy 2025-07-07)/Guidance Test Bench/ControlType/Guidance Testbench/Control Rate Transition ==
  "1 " : Inport
  In2 : Inport  Port=2
  In3 : Inport  Port=3
  In4 : Inport  Port=4
  In5 : Inport  Port=5
  Rate Transition{,1..3} (4 alike) : RateTransition  OutPortSampleTime=ControlSampleTime
  Rate Transition4 : RateTransition  InitialCondition=flightState.Hover  OutPortSampleTime=ControlSampleTime
  Out1 : Outport
  Out2 : Outport  Port=2
  Out3 : Outport  Port=3
  Out4 : Outport  Port=4
  Out5 : Outport  Port=5
  wires:
  In4/1 -> Rate Transition3/1
  In2/1 -> Rate Transition1/1
  Rate Transition4/1 -> Out5/1
  In5/1 -> Rate Transition4/1
  Rate Transition3/1 -> Out4/1
  "1 "/1 -> Rate Transition/1
  Rate Transition1/1 -> Out2/1
  In3/1 -> Rate Transition2/1
  Rate Transition2/1 -> Out3/1
  Rate Transition/1 -> Out1/1

== system VTOLAutopilotController (minhyun-purdue's conflicted copy 2025-07-07)/Guidance Test Bench/ControlType/Guidance Testbench/Guidance Logic ==
  UAVState : Inport
  GCSCommands : Inport  Port=2
  Ground : Inport  Port=3
  Atan2 : Trigonometry  Operator=atan2
  Bus Creator : BusCreator  Inputs=4
  Bus Selector1 : BusSelector  OutputSignals=x,y,z,vy,vx
  Demux : Demux
  Guidance Stateflow : Subsystem
  Interface : Subsystem
  Mux : Mux
  Mux2 : Mux  Inputs=2
  Subsystem : Subsystem
  HoverGuidance : Outport
  FixedWingSP : Outport  Port=2
  AACSP : Outport  Port=3
  ctrlMode : Outport  Port=4
  FlightMode : Outport  Port=5
  wires:
  Mux/1 -> Guidance Stateflow/1(Pose)
  Bus Selector1/5 -> Atan2/2  "<vx>"
  GCSCommands/1 -> Guidance Stateflow/2(GCSCommands)
  Bus Selector1/4 -> Atan2/1  "<vy>"
  Bus Selector1/3 -> Mux2/2, Mux/3  "<z>"
  Bus Selector1/2 -> Mux/2  "<y>"
  UAVState/1 -> Subsystem/1(UAVState), Interface/1(UAVState)
  Bus Selector1/1 -> Mux/1  "<x>"
  Guidance Stateflow/1(HoverCommands) -> Demux/1
  Interface/1(States) -> Bus Selector1/1
  Demux/3 -> Bus Creator/3  "Z"
  Demux/1 -> Bus Creator/1  "X"
  Demux/2 -> Bus Creator/2  "Y"
  Mux2/1 -> Guidance Stateflow/3(LandingStates)
  Atan2/1 -> Mux2/1, Mux/4
  Subsystem/1(States) -> Guidance Stateflow/4(States)
  Guidance Stateflow/3(FixedWingSP) -> FixedWingSP/1
  Guidance Stateflow/2(AACSP) -> AACSP/1
  Guidance Stateflow/4(ctrlMode) -> ctrlMode/1
  Guidance Stateflow/5(FlightMode) -> FlightMode/1
  Bus Creator/1 -> HoverGuidance/1
  Demux/4 -> Bus Creator/4  "Yaw"
  Ground/1 -> Guidance Stateflow/5(Ground)

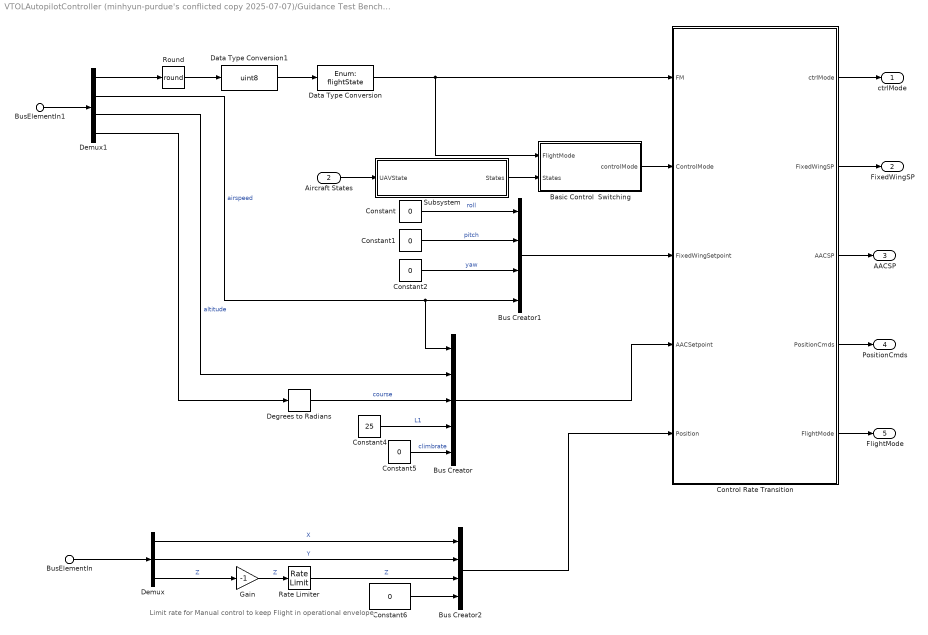
== system VTOLAutopilotController (minhyun-purdue's conflicted copy 2025-07-07)/Guidance Test Bench/ControlType/Manual Control/Command Interface ==
  note: Limit rate for Manual control to keep Flight in operational envelope
  BusElementIn : Inport  PortName=Global Mission  Element=position
  BusElementIn1 : Inport  PortName=Global Mission  Element=params
  Aircraft States : Inport  Port=2
  Basic Control  Switching : Stateflow chart  TreatAsAtomicUnit=on
  Bus Creator : BusCreator  Inputs=5  OutDataTypeStr=Bus: AAC
  Bus Creator1 : BusCreator  Inputs=4  OutDataTypeStr=Bus: FixedWingCommandBus
  Bus Creator2 : BusCreator  Inputs=4
  Constant{,1..2,5..6} (5 alike) : Constant  Value=0
  Constant4 : Constant  Value=25
  Control Rate Transition : Subsystem
  Data Type Conversion : DataTypeConversion  OutDataTypeStr=Enum: flightState  SaturateOnIntegerOverflow=off  RndMeth=Floor
  Data Type Conversion1 : DataTypeConversion  OutDataTypeStr=uint8  SaturateOnIntegerOverflow=off  RndMeth=Floor
  Degrees to Radians : simulink_extras/Transformations/Degrees to Radians
  Demux : Demux  Outputs=3
  Demux1 : Demux
  Gain : Gain  Gain=-1
  Rate Limiter : RateLimiter  RisingSlewLimit=3  FallingSlewLimit=-3  SampleTimeMode=inherited
  Round : Rounding  Operator=round
  Subsystem : Subsystem
  ctrlMode : Outport
  FixedWingSP : Outport  Port=2
  AACSP : Outport  Port=3
  PositionCmds : Outport  Port=4
  FlightMode : Outport  Port=5
  wires:
  Demux1/3 -> Bus Creator/2  "altitude"
  Bus Creator2/1 -> Control Rate Transition/5(Position)
  Constant5/1 -> Bus Creator/5  "climbrate"
  Demux1/4 -> Degrees to Radians/1
  Bus Creator/1 -> Control Rate Transition/4(AACSetpoint)
  Demux/3 -> Gain/1  "Z"
  Data Type Conversion/1 -> Basic Control  Switching/1(FlightMode), Control Rate Transition/1(FM)
  Constant/1 -> Bus Creator1/1  "roll"
  Bus Creator1/1 -> Control Rate Transition/3(FixedWingSetpoint)
  Constant1/1 -> Bus Creator1/2  "pitch"
  Constant4/1 -> Bus Creator/4  "L1"
  Constant2/1 -> Bus Creator1/3  "yaw"
  Demux1/2 -> Bus Creator/1, Bus Creator1/4  "airspeed"
  Control Rate Transition/2(FixedWingSP) -> FixedWingSP/1
  Degrees to Radians/1 -> Bus Creator/3  "course"
  Demux/1 -> Bus Creator2/1  "X"
  Aircraft States/1 -> Subsystem/1(UAVState)
  Demux/2 -> Bus Creator2/2  "Y"
  Gain/1 -> Rate Limiter/1  "Z"
  Basic Control  Switching/1(controlMode) -> Control Rate Transition/2("ControlMode ")
  Control Rate Transition/1(ctrlMode) -> ctrlMode/1
  Control Rate Transition/3(AACSP) -> AACSP/1
  Control Rate Transition/4(PositionCmds) -> PositionCmds/1
  Control Rate Transition/5(FlightMode) -> FlightMode/1
  Demux1/1 -> Round/1
  Subsystem/1(States) -> Basic Control  Switching/2(States)
  Constant6/1 -> Bus Creator2/4
  Rate Limiter/1 -> Bus Creator2/3  "Z"
  BusElementIn/1 -> Demux/1
  BusElementIn1/1 -> Demux1/1
  Round/1 -> Data Type Conversion1/1
  Data Type Conversion1/1 -> Data Type Conversion/1

== system VTOLAutopilotController (minhyun-purdue's conflicted copy 2025-07-07)/Guidance Test Bench/Variant Subsystem/Reference Tracking /Fixed Wing Reference ==
  AAC Commands : Inport
  States : Inport  Port=2
  Bus Creator1 : BusCreator  Inputs=2
  Bus Creator2 : BusCreator  Inputs=3
  Bus Selector : BusSelector  OutputSignals=airspeed,Xe,course
  Bus Selector3 : BusSelector  OutputSignals=airspeed,altitude,course
  Gain : Gain  Gain=-1
  Mux1 : Mux  Inputs=3
  Selector : Selector  InputPortWidth=3  IndexOptions=Index vector (dialog)  Indices=3  OutputSizes=1
  To Workspace1 : ToWorkspace  VariableName=FixedWingCmdFdbk  SaveFormat=Structure With Time  SampleTime=-1
  wires:
  Selector/1 -> Gain/1
  Bus Selector3/1 -> Mux1/1  "<airspeed>"
  Bus Selector/1 -> Bus Creator2/1  "<airspeed>"
  Bus Selector3/2 -> Mux1/2  "<altitude>"
  Bus Selector/3 -> Bus Creator2/3  "<course>"
  Mux1/1 -> Bus Creator1/1
  Bus Creator1/1 -> To Workspace1/1
  Bus Selector3/3 -> Mux1/3  "<course>"
  Gain/1 -> Bus Creator2/2  "altitude"
  Bus Creator2/1 -> Bus Creator1/2
  AAC Commands/1 -> Bus Selector3/1
  Bus Selector/2 -> Selector/1  "<Xe>"
  States/1 -> Bus Selector/1

== system VTOLAutopilotController (minhyun-purdue's conflicted copy 2025-07-07)/Guidance Test Bench/Variant Subsystem/Reference Tracking /Hover Reference ==
  Position Command : Inport
  Position Reference : Inport  Port=2
  Bus Creator : BusCreator  Inputs=2
  Bus Selector1 : BusSelector  OutputSignals=Xe  OutputAsBus=on
  Bus Selector2 : BusSelector  OutputSignals=X,Y,Z
  Mux : Mux  Inputs=3
  To Workspace : ToWorkspace  VariableName=PositionCmdFdbk  SaveFormat=Structure With Time  SampleTime=-1
  wires:
  Position Reference/1 -> Bus Selector1/1
  Bus Selector2/3 -> Mux/3  "<Z>"
  Bus Selector2/1 -> Mux/1  "<X>"
  Bus Selector1/1 -> Bus Creator/2
  Bus Creator/1 -> To Workspace/1
  Bus Selector2/2 -> Mux/2  "<Y>"
  Mux/1 -> Bus Creator/1
  Position Command/1 -> Bus Selector2/1

== system VTOLAutopilotController (minhyun-purdue's conflicted copy 2025-07-07)/Guidance Test Bench/Variant Subsystem/Reference Tracking /Transition Reference ==
  States : Inport
  Bus Creator : BusCreator  Inputs=4
  Bus Selector4 : BusSelector  OutputSignals=airspeed,RotorParameters.Tilt1,Euler,Xe
  Gain : Gain  Gain=-1
  Selector : Selector  InputPortWidth=3  IndexOptions=Index vector (dialog)  Indices=[2]  OutputSizes=1
  Selector1 : Selector  InputPortWidth=3  IndexOptions=Index vector (dialog)  Indices=[3]  OutputSizes=1
  To Workspace1 : ToWorkspace  VariableName=TransitionFeedback  SaveFormat=Structure With Time  SampleTime=-1
  wires:
  States/1 -> Bus Selector4/1
  Bus Selector4/3 -> Selector/1  "<Euler>"
  Bus Selector4/4 -> Selector1/1  "<Xe>"
  Selector1/1 -> Gain/1
  Bus Selector4/1 -> Bus Creator/1  "<airspeed>"
  Selector/1 -> Bus Creator/3  "pitch"
  Gain/1 -> Bus Creator/4  "altitude"
  Bus Creator/1 -> To Workspace1/1
  Bus Selector4/2 -> Bus Creator/2  "<Tilt1>"

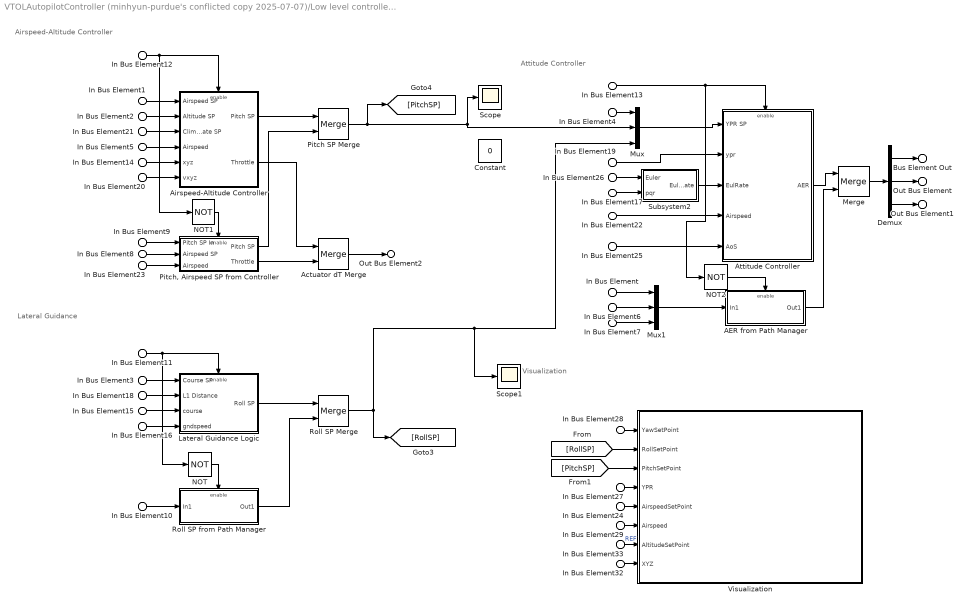
== system VTOLAutopilotController (minhyun-purdue's conflicted copy 2025-07-07)/Low level controller/Fixed Wing Controller/Fixed Wing Controller Module/Fixed Wing Controller Simulation ==
  note: Attitude Controller
  note: Lateral Guidance
  note: Airspeed-Altitude Controller
  note: Visualization
  In Bus Element14 : Inport  PortName=States  Element=Xe
  In Bus Element32 : Inport  PortName=States  Element=Xe
  In Bus Element15 : Inport  PortName=States  Element=course
  In Bus Element17 : Inport  PortName=States  Element=pqr
  In Bus Element{5,22..23,29} (4 alike) : Inport  PortName=States  Element=airspeed
  In Bus Element19 : Inport  PortName=States  Element=ypr
  In Bus Element27 : Inport  PortName=States  Element=ypr
  In Bus Element16 : Inport  PortName=States  Element=gndspeed
  In Bus Element26 : Inport  PortName=States  Element=Euler
  In Bus Element20 : Inport  PortName=States  Element=Ve_ground
  In Bus Element25 : Inport  PortName=States  Element=aos
  In Bus Element11 : Inport  Port=2  PortName=Control Mode  Element=lateralGuidance
  In Bus Element12 : Inport  Port=2  PortName=Control Mode  Element=airspeedAltitude
  In Bus Element13 : Inport  Port=2  PortName=Control Mode  Element=attitude
  In Bus Element1 : Inport  Port=3  PortName=AAC SP  Element=airspeed
  In Bus Element24 : Inport  Port=3  PortName=AAC SP  Element=airspeed
  In Bus Element2 : Inport  Port=3  PortName=AAC SP  Element=altitude
  In Bus Element33 : Inport  Port=3  PortName=AAC SP  Element=altitude
  In Bus Element18 : Inport  Port=3  PortName=AAC SP  Element=L1
  In Bus Element21 : Inport  Port=3  PortName=AAC SP  Element=course
  In Bus Element3 : Inport  Port=3  PortName=AAC SP  Element=course
  In Bus Element4 : Inport  Port=4  PortName=FixedWingSP  Element=yaw
  In Bus Element28 : Inport  Port=4  PortName=FixedWingSP  Element=yaw
  In Bus Element9 : Inport  Port=4  PortName=FixedWingSP  Element=pitch
  In Bus Element10 : Inport  Port=4  PortName=FixedWingSP  Element=roll
  In Bus Element8 : Inport  Port=4  PortName=FixedWingSP  Element=airspeed
  In Bus Element : Inport  Port=5  PortName=AERT  Element=aileron
  In Bus Element6 : Inport  Port=5  PortName=AERT  Element=elevator
  In Bus Element7 : Inport  Port=5  PortName=AERT  Element=rudder
  AER from Path Manager : Subsystem  TreatAsAtomicUnit=on
  Actuator dT Merge : Merge
  Airspeed-Altitude Controller : Subsystem
  Attitude Controller : Subsystem
  Constant : Constant  Value=0
  Demux : Demux  Outputs=3
  Lateral Guidance Logic : Subsystem
  Merge : Merge
  Mux : Mux  Inputs=3
  Mux1 : Mux  Inputs=3
  NOT : Logic  Operator=NOT  IconShape=distinctive  AllPortsSameDT=off  OutDataTypeStr=boolean
  NOT1 : Logic  Operator=NOT  IconShape=distinctive  AllPortsSameDT=off  OutDataTypeStr=boolean
  NOT2 : Logic  Operator=NOT  IconShape=distinctive  AllPortsSameDT=off  OutDataTypeStr=boolean
  Pitch SP Merge : Merge
  "Pitch, Airspeed SP from Controller" : Subsystem  TreatAsAtomicUnit=on
  Roll SP Merge : Merge
  Roll SP from Path Manager : Subsystem  TreatAsAtomicUnit=on
  Scope : Scope
  Scope1 : Scope
  Subsystem2 : Subsystem
  Visualization : Subsystem  Variant=on  VariantControl=Visualization
  Bus Element Out : Outport  PortName=Actuator  Element=dA
  Out Bus Element : Outport  PortName=Actuator  Element=dE
  Out Bus Element1 : Outport  PortName=Actuator  Element=dR
  Out Bus Element2 : Outport  PortName=Actuator  Element=dT
  wires:
  Pitch SP Merge/1 -> Scope/1, Mux/2, [PitchSP]
  Demux/2 -> Out Bus Element/1
  Airspeed-Altitude Controller/1(Pitch SP) -> Pitch SP Merge/1
  In Bus Element18/1 -> Lateral Guidance Logic/2(L1 Distance)
  In Bus Element1/1 -> Airspeed-Altitude Controller/1(Airspeed SP)
  In Bus Element17/1 -> Subsystem2/2(pqr)
  Actuator dT Merge/1 -> Out Bus Element2/1
  In Bus Element26/1 -> Subsystem2/1(Euler)
  In Bus Element11/1 -> Lateral Guidance Logic/Enable, NOT/1
  Subsystem2/1(Euler Rate) -> Attitude Controller/3(EulRate)
  In Bus Element13/1 -> NOT2/1, Attitude Controller/Enable
  In Bus Element3/1 -> Lateral Guidance Logic/1(Course SP)
  In Bus Element22/1 -> Attitude Controller/4(Airspeed)
  Demux/3 -> Out Bus Element1/1
  Roll SP from Path Manager/1(Out1) -> Roll SP Merge/2
  In Bus Element4/1 -> Mux/1
  In Bus Element14/1 -> Airspeed-Altitude Controller/5(xyz)
  In Bus Element15/1 -> Lateral Guidance Logic/3(course)
  In Bus Element6/1 -> Mux1/2
  Mux1/1 -> AER from Path Manager/1(In1)
  Airspeed-Altitude Controller/2(Throttle) -> Actuator dT Merge/1
  "Pitch, Airspeed SP from Controller"/1(Pitch SP) -> Pitch SP Merge/2
  In Bus Element16/1 -> Lateral Guidance Logic/4(gndspeed)
  "Pitch, Airspeed SP from Controller"/2(Throttle) -> Actuator dT Merge/2
  In Bus Element/1 -> Mux1/1
  In Bus Element2/1 -> Airspeed-Altitude Controller/2(Altitude SP)
  In Bus Element7/1 -> Mux1/3
  In Bus Element9/1 -> "Pitch, Airspeed SP from Controller"/1(Pitch SP In)
  Merge/1 -> Demux/1
  In Bus Element10/1 -> Roll SP from Path Manager/1(In1)
  Mux/1 -> Attitude Controller/1(YPR SP)
  Attitude Controller/1(AER) -> Merge/1
  NOT1/1 -> "Pitch, Airspeed SP from Controller"/Enable
  In Bus Element8/1 -> "Pitch, Airspeed SP from Controller"/2(Airspeed SP)
  In Bus Element20/1 -> Airspeed-Altitude Controller/6(vxyz)
  In Bus Element19/1 -> Attitude Controller/2(ypr)
  NOT2/1 -> AER from Path Manager/Enable
  In Bus Element23/1 -> "Pitch, Airspeed SP from Controller"/3(Airspeed)
  Lateral Guidance Logic/1(Roll SP) -> Roll SP Merge/1
  NOT/1 -> Roll SP from Path Manager/Enable
  AER from Path Manager/1(Out1) -> Merge/2
  In Bus Element5/1 -> Airspeed-Altitude Controller/4(Airspeed)
  Demux/1 -> Bus Element Out/1
  In Bus Element21/1 -> Airspeed-Altitude Controller/3(Climb Rate SP)
  Roll SP Merge/1 -> [RollSP], Scope1/1, Mux/3
  In Bus Element12/1 -> Airspeed-Altitude Controller/Enable, NOT1/1
  In Bus Element28/1 -> Visualization/1(YawSetPoint)
  In Bus Element27/1 -> Visualization/4(YPR)
  In Bus Element24/1 -> Visualization/5(AirspeedSetPoint)
  In Bus Element29/1 -> Visualization/6(Airspeed)
  In Bus Element33/1 -> Visualization/7(AltitudeSetPoint)  "REF"
  In Bus Element32/1 -> Visualization/8(XYZ)
  [RollSP] -> Visualization/2(RollSetPoint)
  [PitchSP] -> Visualization/3(PitchSetPoint)
  In Bus Element25/1 -> Attitude Controller/5(AoS)
